simulink model "IMDriveSensor00"  (R2025a)
settings: Solver=FixedStepAuto  StartTime=0.0  StopTime=25  FixedStep=Ts  MaxStep=1e-3  RelTol=1e-3  EnableMultiTasking=on
PreLoadFcn:
  | IMDriveSensorData
values from neighbouring files (symbols this model uses):
  fn = 50    [IMDriveSensorData.m]
  Ibase = Pn/(1.5*Vbase)    [IMDriveSensorData.m]
  It1base = Pt/(1.5*Vt1base)    [IMDriveSensorData.m]
  Ki_id = 17.64    [IMDriveSensorData.m]
  Ki_ids = 207.58    [IMDriveSensorData.m]
  Ki_imr = 2790.51    [IMDriveSensorData.m]
  Ki_iq = 20.81    [IMDriveSensorData.m]
  Ki_iqs = 210.02    [IMDriveSensorData.m]
  Ki_vdc = 681.12    [IMDriveSensorData.m]
  Ki_wr = 3134.24    [IMDriveSensorData.m]
  Kp_id = 0.84    [IMDriveSensorData.m]
  Kp_ids = 1.08    [IMDriveSensorData.m]
  Kp_imr = 52.22    [IMDriveSensorData.m]
  Kp_iq = 0.99    [IMDriveSensorData.m]
  Kp_iqs = 1.08    [IMDriveSensorData.m]
  Kp_vdc = 3.54    [IMDriveSensorData.m]
  Kp_wr = 65.47    [IMDriveSensorData.m]
  Leq = (L1 + L2*(V1/V2)^2)/(Zt1base/wtbase)    [IMDriveSensorData.m]
  Lm = 1.36    [IMDriveSensorData.m]
  N = V2/V1    (= 1)    [IMDriveSensorData.m]
  p = 2    [IMDriveSensorData.m]
  Req = (R1 + R2*(V1/V2)^2)/Zt1base    [IMDriveSensorData.m]
  Tbase = Pn/(wbase/p)    (= 3.56507072526)    [IMDriveSensorData.m]
  Ts = 5e-6    (= 5e-06)    [IMDriveSensorData.m]
  Tsc = 1/(fsw*10)    (= 5e-05)    [IMDriveSensorData.m]
  Vbase = Vn/sqrt(3)*sqrt(2)    [IMDriveSensorData.m]
  Vt1base = V1/sqrt(3)*sqrt(2)    [IMDriveSensorData.m]
  wtbase = 2*pi*ft    (= 314.159265359)    [IMDriveSensorData.m]
  Xls = Lls*Zbase    [IMDriveSensorData.m]
undefined symbols (not defined in the file or in its folder): ee
libraries: nesl_utility x23, ee_lib x16, fl_lib x8, slpidlib x7, eeTransforms x4, eeGeneralControl x4, simulink x3, eePwmGeneratorTwoLevel x2, eeSinusoidalMeasurement x1, eeAsmFluxObserver x1, spsPLL3phLib x1
(part 1 of 2)
CloseFcn:
  | clear simlog_IMDriveSensor
  | clear logsout_IMDriveSensor
Description:
  | Three-Phase Asynchronous Drive with Sensor Control
settings Model: Creator=The MathWorks, Inc.  LastModifiedBy=vhovh
settings SolverCC: AlgebraicLoopSolver=TrustRegion  AutoInsertRateTranBlk=on
settings DataIOCC: MaxDataPoints=510000  SaveOperatingPoint=on  SaveFormat=StructureWithTime  SaveOutput=off  SaveTime=off  ReturnWorkspaceOutputs=off  SignalLoggingName=logsout_IMDriveSensor
settings OptimizationCC: ReuseModelBlockBuffer=off  ExpressionDepthLimit=2147483647.0  LifeSpan=inf
settings DebuggingCC: AlgebraicLoopMsg=error  UnderspecifiedInitializationDetection=Classic  MergeDetectMultiDrivingBlocksExec=none  SolverPrmCheckMsg=warning  MultiTaskRateTransMsg=warning  UnconnectedInputMsg=warning  UnconnectedOutputMsg=warning  UnconnectedLineMsg=warning  StateNameClashWarn=warning  SFUnexpectedBacktrackingDiag=warning  SFNoUnconditionalDefaultTransitionDiag=warning  SFExecutionAtInitializationDiag=none  ArithmeticOperatorsInVariantConditions=warning
settings HardwareCC: ProdBitPerPointer=32.0  ProdBitPerSizeT=32.0  ProdBitPerPtrDiffT=32.0  ProdLargestAtomicFloat=None  ProdIntDivRoundTo=Undefined  ProdEndianess=Unspecified  ProdWordSize=32.0  ProdHWDeviceType=32-bit Generic
settings ModelReferenceCC: EnableRefExpFcnMdlSchedulingChecks=on  PropagateSignalLabelsOutOfModel=off
settings SFSimCC: SimUseLocalCustomCode=off  CustomCodeUndefinedFunction=UseInterfaceOnly
settings RTWCC: RTWUseLocalCustomCode=off  GPUComputeCapability=3.5  DLArmComputeVersion=19.05
settings CodeAppCC: StateflowObjectComments=on
settings GRTTargetCC: TargetLangStandard=C89/C90 (ANSI)
settings ConfigComp: CovMetricSettings=dw  CovSaveCumulativeToWorkspaceVar=on  CovSaveSingleToWorkspaceVar=on  CovExternalEMLEnable=off  CovSFcnEnable=off
settings SimscapeCC: SimscapeLogType=all  SimscapeLogSimulationStatistics=on  SimscapeLogName=simlog_IMDriveSensor  SimscapeLogDecimation=5.0  SimscapeLogDataHistory=510000.0

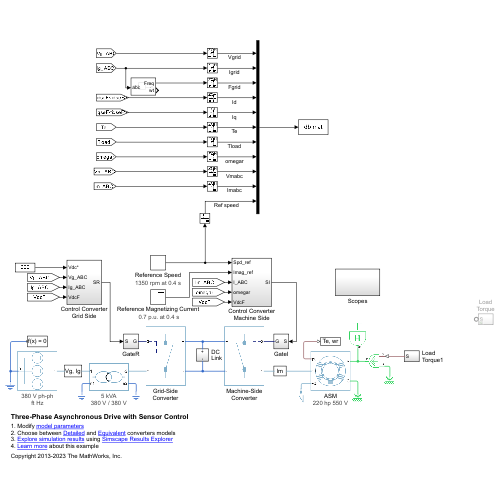
[thumbnail: Simulink's stored preview of the top-level diagram]
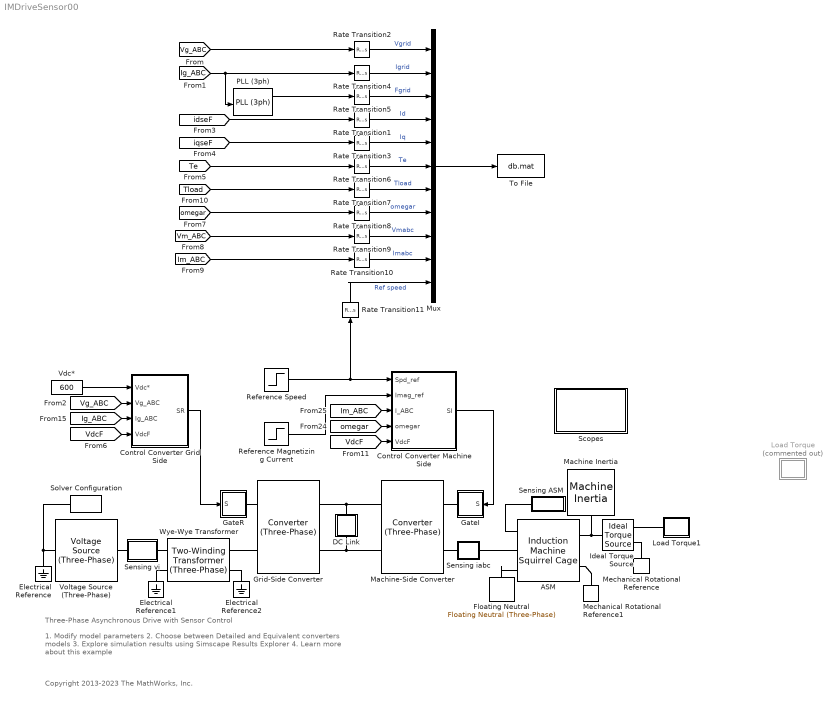
== system IMDriveSensor00 ==
  note: 1. Modify model parameters
      | 2. Choose between Detailed and Equivalent converters models
      | 3. Explore simulation results using Simscape Results Explorer
      | 4. Learn more about this example
  note: Three-Phase Asynchronous Drive with Sensor Control
  note: Copyright 2013-2023 The MathWorks, Inc.
  ASM : ee_lib/Electromechanical/Asynchronous/Induction Machine Squirrel Cage  port_option=ee.enum.threePhasePort.composite  SRated=Pn V*A  VRated=Vn V  FRated=fn Hz  nPolePairs=p  param_unit=ee.enum.unit.si  squirrel_cage=ee.enum.squirrelcage.Single  zero_sequence=ee.enum.park.zerosequence.include  initialization_option=ee.enum.asm.initialization.fluxvariables  Rs=Rss Ohm  Xls=Xls Ohm  pu_Rs=0.039  pu_Lls=0.194  Rrd=Rrr Ohm  Xlrd=Xlr Ohm  pu_Rrd=0.031  pu_Llrd=0.194  Rrd1=0.28 Ohm  Xlrd1=0.82 Ohm  Rrd2=0.28 Ohm  Xlrd2=0.82 Ohm  pu_Rrd1=0.0290  pu_Llrd1=0.0848  pu_Rrd2=0.0290  pu_Llrd2=0.0848  Xm=Xm Ohm  pu_Lm=1.36  X0=Xls Ohm  pu_L0=0.194  saturation_option=0  saturation_i=[0, 4, 9, 18, 25, 34, 50, 68, 95, 120] A  saturation_v=[0, 88, 154, 198, 220, 242, 264, 286, 308, 330] V  pu_saturation_i=[0, .176, .396, .792, 1.1, 1.496, 2.2, 2.992, 4.18, 5.28]  pu_saturation_v=[0, .4, .7, .9, 1, 1.1, 1.2, 1.3, 1.4, 1.4864]  connection_option=int32(ee.enum.Connection.delta)  angular_position_specify=off  angular_position_priority=None  angular_position=0 deg  angular_position_nominal_specify=off  angular_position_nominal_value=1  angular_position_nominal_unit=deg  pu_psids_specify=off  pu_psids_priority=None  pu_psids=0  pu_psids_nominal_specify=off  pu_psids_nominal_value=1  pu_psids_nominal_unit=1  pu_psiqs_specify=off  pu_psiqs_priority=None  pu_psiqs=0  pu_psiqs_nominal_specify=off  pu_psiqs_nominal_value=1  pu_psiqs_nominal_unit=1  pu_psi0s_specify=off  pu_psi0s_priority=None  pu_psi0s=0  pu_psi0s_nominal_specify=off  pu_psi0s_nominal_value=1  pu_psi0s_nominal_unit=1  pu_psidr_specify=off  pu_psidr_priority=None  pu_psidr=0  pu_psidr_nominal_specify=off  pu_psidr_nominal_value=1  pu_psidr_nominal_unit=1  pu_psiqr_specify=off  pu_psiqr_priority=None  pu_psiqr=0  pu_psiqr_nominal_specify=off  pu_psiqr_nominal_value=1  pu_psiqr_nominal_unit=1  pu_psidr1_specify=off  pu_psidr1_priority=None  pu_psidr1=0  pu_psidr1_nominal_specify=off  pu_psidr1_nominal_value=1  pu_psidr1_nominal_unit=1  pu_psiqr1_specify=off  pu_psiqr1_priority=None  pu_psiqr1=0  pu_psiqr1_nominal_specify=off  pu_psiqr1_nominal_value=1  pu_psiqr1_nominal_unit=1  pu_psidr2_specify=off  pu_psidr2_priority=None  pu_psidr2=0  pu_psidr2_nominal_specify=off  pu_psidr2_nominal_value=1  pu_psidr2_nominal_unit=1  pu_psiqr2_specify=off  pu_psiqr2_priority=None  pu_psiqr2=0  pu_psiqr2_nominal_specify=off  pu_psiqr2_nominal_value=1  pu_psiqr2_nominal_unit=1  psids_specify=off  psids_priority=None  psids=0 Wb  psids_nominal_specify=off  psids_nominal_value=1  psids_nominal_unit=Wb  psiqs_specify=off  psiqs_priority=None  psiqs=0 Wb  psiqs_nominal_specify=off  psiqs_nominal_value=1  psiqs_nominal_unit=Wb  psi0s_specify=off  psi0s_priority=None  psi0s=0 Wb  psi0s_nominal_specify=off  psi0s_nominal_value=1  psi0s_nominal_unit=Wb  psidr_specify=off  psidr_priority=None  psidr=0 Wb  psidr_nominal_specify=off  psidr_nominal_value=1  psidr_nominal_unit=Wb  psiqr_specify=off  psiqr_priority=None  psiqr=0 Wb  psiqr_nominal_specify=off  psiqr_nominal_value=1  psiqr_nominal_unit=Wb  psidr1_specify=off  psidr1_priority=None  psidr1=0 Wb  psidr1_nominal_specify=off  psidr1_nominal_value=1  psidr1_nominal_unit=Wb  psiqr1_specify=off  psiqr1_priority=None  psiqr1=0 Wb  psiqr1_nominal_specify=off  psiqr1_nominal_value=1  psiqr1_nominal_unit=Wb  psidr2_specify=off  psidr2_priority=None  psidr2=0 Wb  psidr2_nominal_specify=off  psidr2_nominal_value=1  psidr2_nominal_unit=Wb  psiqr2_specify=off  psiqr2_priority=None  psiqr2=0 Wb  psiqr2_nominal_specify=off  psiqr2_nominal_value=1  psiqr2_nominal_unit=Wb  slip_specify=off  slip_priority=None  slip=0  slip_nominal_specify=off  slip_nominal_value=1  slip_nominal_unit=1  real_power_generated_specify=off  real_power_generated_priority=None  real_power_generated=0 W  real_power_generated_nominal_specify=off  real_power_generated_nominal_value=1  real_power_generated_nominal_unit=W  mechanical_power_consumed_specify=off  mechanical_power_consumed_priority=None  mechanical_power_consumed=0 W  mechanical_power_consumed_nominal_specify=off  mechanical_power_consumed_nominal_value=1  mechanical_power_consumed_nominal_unit=W  Tmeas=298.15 K  alpha=3.93e-3 1/K  alpha_cage=4.4e-3 1/K  stator_thermal_mass=100 J/K  rotor_thermal_mass=200 J/K  temperatureA_specify=off  temperatureA_priority=High  temperatureA=25 degC  temperatureA_nominal_specify=off  temperatureA_nominal_value=1  temperatureA_nominal_unit=degC  temperatureB_specify=off  temperatureB_priority=High  temperatureB=25 degC  temperatureB_nominal_specify=off  temperatureB_nominal_value=1  temperatureB_nominal_unit=degC  temperatureC_specify=off  temperatureC_priority=High  temperatureC=25 degC  temperatureC_nominal_specify=off  temperatureC_nominal_value=1  temperatureC_nominal_unit=degC  temperatureR_specify=off  temperatureR_priority=High  temperatureR=25 degC  temperatureR_nominal_specify=off  temperatureR_nominal_value=1  temperatureR_nominal_unit=degC
      settings: AttributesFormatString=220 hp 550 V  InternalSimscapePortConfiguration="{\"Bottom\":[],\"Left\":[{\"id\":\"R\",\"label\":\"R\",\"type\":\"foundation.mechanical.rotational.rotational\"},{\"id\":\"C\",\"label\":\"C\",\"type\":\"foundation.mechanical.rotational.rotational\"}],\"Right\":[{\"id\":\"pu_output\",\"label\":\"pu\",\"type\":\"output\"},{\"id\":\"N1\",\"label\":\"~1\",\"type\":\"foundation.electrical.three_phase\"},{\"id\":\"N2\",\"label\":\"~2\",\"type\":\"foundation.electrical.three_phase\"}],\"Top\":[]}"
  Control Converter Grid Side : Subsystem
  Control Converter Machine Side : Subsystem
  DC Link : Subsystem
  Electrical Reference : fl_lib/Electrical/Electrical Elements/Electrical Reference
  Electrical Reference1 : fl_lib/Electrical/Electrical Elements/Electrical Reference
  Electrical Reference2 : fl_lib/Electrical/Electrical Elements/Electrical Reference
  Floating Neutral : ee_lib/Connectors & References/Floating Neutral (Three-Phase)  G_parasitic=1e-12 1/Ohm
      settings: InternalSimscapePortConfiguration="{\"Bottom\":[],\"Left\":[{\"id\":\"N\",\"label\":\"~\",\"type\":\"foundation.electrical.three_phase\"}],\"Right\":[],\"Top\":[]}"
  GateI : Subsystem
  GateR : Subsystem
  Grid-Side Converter : ee_lib/Semiconductors & Converters/Converters/Converter (Three-Phase)  port_option=ee.enum.threePhasePort.composite  fidelity_option=ee.enum.converters.fidelity.equivalent_pwm  device_type=3  showThermalPort=false  K=0  Vth=0.5 V  Vgt=1 V  Vgt_off=-1 V  Ih=1 A  Vf=0.8 V  Ron=0.001 Ohm  Rds=0.001 Ohm  Goff=1e-5 1/Ohm  Eon_scalar=22.86e-3 J  Eoff_scalar=17.14e-3 J  Eoff_natural_commutation=10e-3 J  Voff=300 V  Iout_scalar=600 A  onCurrentMeasDelay=0 s  useCurrentFromPreviousCycle=false  useVoltageFromPreviousCycle=false  diode_param=2  diode_Vf=0.8 V  diode_Ron=0.001 Ohm  diode_Goff=1e-5 1/Ohm  diode_C=50 nF  diode_iRM=-235 A  diode_iF=300 A  diode_idot=-50 A/us  diode_trr_param=1  diode_trr_factor=3  diode_trr=15 us  diode_Qrr=1.5e+3 s*uA  diode_rec_loss_model=ee.enum.diode.reverseRecoveryModel.fixed  diode_ErecVal=0 J  diode_scaleWithIandV=false  diode_ErecMat=zeros(2, 3) J  diode_TjrecVec=[298.15, 398.15] K  diode_IfrecVec=[.1, 1, 10] A  diode_IrecVal=10 A  diode_VrecVal=10 V  diode_tFilter=1 / 1000 / 100 s  thermal_network_parameterization=ee.enum.thermalNetworkTopology.external  Rth=[.08, .5] K/W  Rth_Cauer=[.08, .1, .5] K/W  Rth_Foster=[.08, .14, .22, .16] K/W  thermal_mass_parameterization=ee.enum.thermalNetwork.timeconstant  thermal_mass=[.01, .5] J/K  thermal_mass_Cauer=[.01, .1, .5] J/K  thermal_mass_Foster=[.001, .005, .05, .5] J/K  thermal_time_constant=[.001, .2] s  thermal_time_constant_Cauer=[.001, .1, .2] s  thermal_time_constant_Foster=[7e-05, .0007, .01, .08] s  thermal_mass_initial_temperatures=[25, 25] degC  thermal_mass_initial_temperatures_Cauer=[25, 25, 25] degC  junction_thermal_mass=0.01 J/K  Tvec_initial_Foster=[25, 25, 25, 25] degC  snubber_type=0  Cs=1e-5 F  Rs=1e-3 Ohm  Vce_loss=[0, 150, 300] V
  Ideal Torque Source : fl_lib/Mechanical/Mechanical Sources/Ideal Torque Source
  Load Torque : Subsystem  Commented=on
  Load Torque1 : Subsystem
  Machine Inertia : ee_lib/Electromechanical/Mechanical/Machine Inertia  SRated=Pn V*A  FRated=fn Hz  nPolePairs=p  inertia_option=2  J=27548 kg*m^2  H=H s*W/V/A  damper_option=2  D=39.0509 N*m/(rad/s)  pu_D=F  initialization_option=2  fMechanical0=60 Hz  fElectrical0=0 Hz
      settings: InternalSimscapePortConfiguration="{\"Bottom\":[],\"Left\":[{\"id\":\"R\",\"label\":\"R\",\"type\":\"foundation.mechanical.rotational.rotational\"}],\"Right\":[],\"Top\":[]}"
  Machine-Side Converter : ee_lib/Semiconductors & Converters/Converters/Converter (Three-Phase)  port_option=ee.enum.threePhasePort.composite  fidelity_option=ee.enum.converters.fidelity.equivalent_pwm  device_type=3  showThermalPort=false  K=0  Vth=0.5 V  Vgt=1 V  Vgt_off=-1 V  Ih=1 A  Vf=0.8 V  Ron=0.001 Ohm  Rds=0.001 Ohm  Goff=1e-5 1/Ohm  Eon_scalar=22.86e-3 J  Eoff_scalar=17.14e-3 J  Eoff_natural_commutation=10e-3 J  Voff=300 V  Iout_scalar=600 A  onCurrentMeasDelay=0 s  useCurrentFromPreviousCycle=false  useVoltageFromPreviousCycle=false  diode_param=2  diode_Vf=0.8 V  diode_Ron=0.001 Ohm  diode_Goff=1e-5 1/Ohm  diode_C=50 nF  diode_iRM=-235 A  diode_iF=300 A  diode_idot=-50 A/us  diode_trr_param=1  diode_trr_factor=3  diode_trr=15 us  diode_Qrr=1.5e+3 s*uA  diode_rec_loss_model=ee.enum.diode.reverseRecoveryModel.fixed  diode_ErecVal=0 J  diode_scaleWithIandV=false  diode_ErecMat=zeros(2, 3) J  diode_TjrecVec=[298.15, 398.15] K  diode_IfrecVec=[.1, 1, 10] A  diode_IrecVal=10 A  diode_VrecVal=10 V  diode_tFilter=1 / 1000 / 100 s  thermal_network_parameterization=ee.enum.thermalNetworkTopology.external  Rth=[.08, .5] K/W  Rth_Cauer=[.08, .1, .5] K/W  Rth_Foster=[.08, .14, .22, .16] K/W  thermal_mass_parameterization=ee.enum.thermalNetwork.timeconstant  thermal_mass=[.01, .5] J/K  thermal_mass_Cauer=[.01, .1, .5] J/K  thermal_mass_Foster=[.001, .005, .05, .5] J/K  thermal_time_constant=[.001, .2] s  thermal_time_constant_Cauer=[.001, .1, .2] s  thermal_time_constant_Foster=[7e-05, .0007, .01, .08] s  thermal_mass_initial_temperatures=[25, 25] degC  thermal_mass_initial_temperatures_Cauer=[25, 25, 25] degC  junction_thermal_mass=0.01 J/K  Tvec_initial_Foster=[25, 25, 25, 25] degC  snubber_type=0  Cs=1e-7 F  Rs=0.1 Ohm  Vce_loss=[0, 150, 300] V
  Mechanical Rotational Reference : fl_lib/Mechanical/Rotational Elements/Mechanical Rotational Reference
  Mechanical Rotational Reference1 : fl_lib/Mechanical/Rotational Elements/Mechanical Rotational Reference
  Mux : Mux  Inputs=11
  PLL (3ph) : spsPLL3phLib/PLL (3ph)  Fmin=45  Par_Init=[0, 60]  ParK=[180, 3200, 1]  TcD=1e-4  MaxRateChangeFreq=12  FilterCutOffFreq=25  Ts=0  AGC=on
  Rate Transition{1..11} (11 alike) : RateTransition  OutPortSampleTime=0.1
  Reference Magnetizing Current : Step  Time=0.4  After=0.7*1/Lm  SampleTime=Tsc
      settings: AttributesFormatString=0.7 p.u. at 0.4 s
  Reference Speed : Step  Time=0.4  After=1350  SampleTime=Tsc
      settings: AttributesFormatString=%<After> rpm at %<Time> s
  Scopes : Subsystem
  Sensing ASM : Subsystem
      mask Display: disp('Te, wr')
  Sensing iabc : Subsystem
      mask Display: disp('Im')
  Sensing vi : Subsystem
      mask Display: disp('Vg, Ig')
  Solver Configuration : nesl_utility/Solver Configuration  PhysicalDomain=network_engine_domain  SubClassName=solver  LeftPortType=input  RightPortType=generic  Tones=[]  Harmonics=[]  SimulateNoise=off  Profile=off  UseLocalSampling=off  EnableSwitchedLinearOptims=on  FrequencyDomain=off  UseCCode=off  RelTol=0.001  AbsTol=1e-06  MinStep=1e-09  ToWorkspace=off  RevertToSquareIcSolve=off  NumHomotopyIterations=100  PhasorMode=off  PhasorModeNumHarmonics=1  ConsistencySolver=NEWTON_FTOL  IndexReductionMethod=DerivativeReplacement  DoDC=off  ResidualTolerance=1e-09  ConsistencyTolSource=GLOBAL  ConsistencyAbsTol=0.001  ConsistencyRelTol=0.001  ConsistencyTolFactor=0.001  UseLocalSolver=on  LocalSolverChoice=NE_BACKWARD_EULER_ADVANCER  ResolveIndetEquations=on  FunctionEvalNumThread=1  LocalSolverSampleTime=Ts  DoFixedCost=on  MaxNonlinIter=5  MaxModeIter=2  ComputeImpulses=off  ImpulseIterations=2  LinearAlgebra=auto  LinearAlgebraNumThread=0  EquationFormulation=NE_TIME_EF  DelaysMemoryBudget=1024  AutomaticFiltering=on  FilteringTimeConstant=0.001  PartitionStorageMethod=AS_NEEDED  PartitionMemoryBudget=1024  PartitionMethod=FAST  MultibodyUseLocalSolver=off  MultibodyLocalSolverChoice=ODE1  MultibodyLocalSolverSampleTime=0.001
  To File : ToFile  Filename=db.mat  SaveFormat=Timeseries
  Vdc* : Constant  Value=600
  Voltage Source (Three-Phase) : ee_lib/Sources/Voltage Source (Three-Phase)  vline_rms=380 V  shift=0 deg  freq=ft Hz  impedance_option=0  SShortCircuit=1e6 V*A  XR=15  R=0.01 Ohm  L=3.97e-4 H  harmonic_option=0  harmonic_orders=[5.0, 7.0, 11.0, 13.0]  harmonic_ratios=[0.1, 0.1, 0.1, 0.1]  G_parasitic=0 1/Ohm  I_specify=off  I_priority=None  I=[ 0 0 0 ] A  I_nominal_specify=off  I_nominal_value=1  I_nominal_unit=A
      settings: AttributesFormatString=|
      | %<vline_rms> %<vline_rms_unit> ph-ph
      | %<freq> %<freq_unit>
  Wye-Wye Transformer : ee_lib/Passive/Transformers/Two-Winding Transformer (Three-Phase)  SRated=Pt V*A  FRated=ft Hz  Winding1Connection=ee.enum.windingconnection.Yn  VRated1=V1 V  Winding2Connection=ee.enum.windingconnection.Yn  VRated2=V2 V  CoreType=ee.enum.coretype.threelimb  pu_Rw1=0.01  pu_Rw2=0.01  leakage_reactance_option=ee.enum.transformer_leakage.include  pu_Xl1=L1pu  pu_Xl2=L2pu  magnetizing_resistance_option=ee.enum.transformer_magnetizingResistance.include  pu_Rm=500  magnetizing_reactance_option=ee.enum.transformer_magnetizingReactance.include  saturation_option=ee.enum.transformer_saturation.exclude  pu_Xm=500  current_data=[0, .002, 1, 2]  magnetic_flux_data=[0, 1.2, 1.5, 1.51]  pu_X0=0.5  i1_specify=off  i1_priority=None  i1=[ 0 0 0 ] A  i1_nominal_specify=off  i1_nominal_value=1  i1_nominal_unit=A  i2_specify=off  i2_priority=None  i2=[ 0 0 0 ] A  i2_nominal_specify=off  i2_nominal_value=1  i2_nominal_unit=A  phi_specify=off  phi_priority=None  phi=[ 0 0 0 ]  phi_nominal_specify=off  phi_nominal_value=1  phi_nominal_unit=1  power_dissipated_specify=off  power_dissipated_priority=None  power_dissipated=0 W  power_dissipated_nominal_specify=off  power_dissipated_nominal_value=1  power_dissipated_nominal_unit=W
      settings: InternalSimscapePortConfiguration="{\"Bottom\":[],\"Left\":[{\"id\":\"N1\",\"label\":\"~1\",\"type\":\"foundation.electrical.three_phase\"},{\"id\":\"n1\",\"label\":\"n1\",\"type\":\"foundation.electrical.electrical\"}],\"Right\":[{\"id\":\"N2\",\"label\":\"~2\",\"type\":\"foundation.electrical.three_phase\"},{\"id\":\"n2\",\"label\":\"n2\",\"type\":\"foundation.electrical.electrical\"}],\"Top\":[]}"
      settings: AttributesFormatString=|
      | 5 kVA
      | 380 V / 380 V
  wires:
  Control Converter Grid Side/1(SR) -> GateR/1(S)
  Control Converter Machine Side/1(SI) -> GateI/1(S)
  Reference Speed/1 -> Rate Transition11/1, Control Converter Machine Side/1(Spd_ref)
  Reference Magnetizing Current/1 -> Control Converter Machine Side/2(Imag_ref)
  Vdc*/1 -> Control Converter Grid Side/1(Vdc*)
  [Vg_ABC] -> Control Converter Grid Side/2(Vg_ABC)
  [Ig_ABC] -> Control Converter Grid Side/3(Ig_ABC)
  [VdcF] -> Control Converter Grid Side/4(VdcF)
  [Im_ABC] -> Control Converter Machine Side/3(I_ABC)
  [omegar] -> Control Converter Machine Side/4(omegar)
  [VdcF] -> Control Converter Machine Side/5(VdcF)
  [Vg_ABC] -> Rate Transition2/1
  [Ig_ABC] -> PLL (3ph)/1, Rate Transition4/1
  PLL (3ph)/1 -> Rate Transition5/1
  [Te] -> Rate Transition6/1
  [Tload] -> Rate Transition7/1
  [omegar] -> Rate Transition8/1
  [Vm_ABC] -> Rate Transition9/1
  [Im_ABC] -> Rate Transition10/1
  Mux/1 -> To File/1
  [iqseF] -> Rate Transition3/1
  [idseF] -> Rate Transition1/1
  Rate Transition2/1 -> Mux/1  "Vgrid"
  Rate Transition4/1 -> Mux/2  "Igrid"
  Rate Transition5/1 -> Mux/3  "Fgrid"
  Rate Transition1/1 -> Mux/4  "Id"
  Rate Transition3/1 -> Mux/5  "Iq"
  Rate Transition6/1 -> Mux/6  "Te"
  Rate Transition7/1 -> Mux/7  "Tload"
  Rate Transition8/1 -> Mux/8  "omegar"
  Rate Transition9/1 -> Mux/9  "Vmabc"
  Rate Transition10/1 -> Mux/10  "Imabc"
  Rate Transition11/1 -> Mux/11  "Ref speed"
  connections:
  Electrical Reference/LConn1 -- Solver Configuration/RConn1 -- Voltage Source (Three-Phase)/LConn1
  Sensing vi/LConn1 -- Voltage Source (Three-Phase)/RConn1
  Sensing vi/RConn1 -- Wye-Wye Transformer/LConn1
  Electrical Reference1/LConn1 -- Wye-Wye Transformer/LConn2
  Wye-Wye Transformer/RConn2 -- Electrical Reference2/LConn1
  Grid-Side Converter/LConn2 -- Wye-Wye Transformer/RConn1
  Grid-Side Converter/RConn1 -- DC Link/LConn1 -- Machine-Side Converter/RConn1
  Grid-Side Converter/RConn2 -- DC Link/RConn1 -- Machine-Side Converter/RConn2
  Sensing iabc/LConn1 -- Machine-Side Converter/LConn2
  ASM/RConn2 -- Sensing iabc/RConn1
  ASM/LConn1 -- Machine Inertia/LConn1 -- Ideal Torque Source/LConn1
  Mechanical Rotational Reference/LConn1 -- Ideal Torque Source/RConn2
  GateR/RConn1 -- Grid-Side Converter/LConn1
  GateI/RConn1 -- Machine-Side Converter/LConn1
  Floating Neutral/LConn1 -- ASM/RConn3
  Mechanical Rotational Reference1/LConn1 -- ASM/LConn2
  Load Torque1/RConn1 -- Ideal Torque Source/RConn1
  ASM/RConn1 -- Sensing ASM/RConn1

== system IMDriveSensor00/Control Converter Grid Side ==
  Vdc* : Inport
  Vg_ABC : Inport  Port=2
  Ig_ABC : Inport  Port=3
  VdcF : Inport  Port=4
  Control : Subsystem
  Measurements : Subsystem
  SR : Outport  VectorParamsAs1DForOutWhenUnconnected=off
  wires:
  Vdc*/1 -> Control/1(Vdc)
  VdcF/1 -> Control/2(VdcF)
  Control/1(SR) -> SR/1
  Vg_ABC/1 -> Measurements/1(Vg_ABC)
  Ig_ABC/1 -> Measurements/2(Ig_ABC)
  Measurements/1(omega) -> Control/3(omega)
  Measurements/2(Vg) -> Control/4(Vg)
  Measurements/3(idF) -> Control/5(idF)
  Measurements/4(theta) -> Control/6(theta)
  Measurements/5(iqF) -> Control/7(iqF)

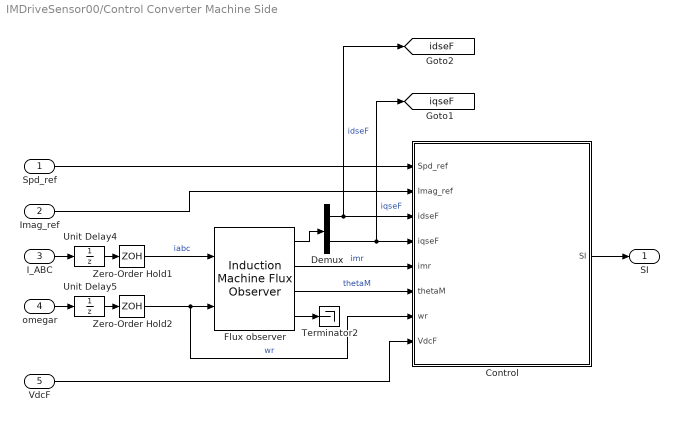
== system IMDriveSensor00/Control Converter Machine Side ==
  Spd_ref : Inport
  Imag_ref : Inport  Port=2
  I_ABC : Inport  Port=3
  omegar : Inport  Port=4
  VdcF : Inport  Port=5
  Control : Subsystem
  Demux : Demux  Outputs=2
  Flux observer : eeAsmFluxObserver/Induction Machine Flux Observer  fn=fn  Rr=Rr  Llr=Llr  Lm=Lm  Tc=1e-4  Ts=Tsc
  Terminator2 : Terminator
  Unit Delay4 : UnitDelay  SampleTime=Ts  HasFrameUpgradeWarning=on
  Unit Delay5 : UnitDelay  SampleTime=Ts  HasFrameUpgradeWarning=on
  Zero-Order Hold1 : ZeroOrderHold  SampleTime=Tsc
  Zero-Order Hold2 : ZeroOrderHold  SampleTime=Tsc
  SI : Outport  VectorParamsAs1DForOutWhenUnconnected=off
  tag scope: idseF=global, iqseF=global
  wires:
  Zero-Order Hold1/1 -> Flux observer/1  "iabc"
  Flux observer/1 -> Demux/1
  Flux observer/4 -> Terminator2/1
  Imag_ref/1 -> Control/2(Imag_ref)
  Demux/1 -> [idseF], Control/3(idseF)  "idseF"
  Demux/2 -> [iqseF], Control/4(iqseF)  "iqseF"
  Flux observer/2 -> Control/5(imr)  "imr"
  Flux observer/3 -> Control/6(thetaM)  "thetaM"
  Zero-Order Hold2/1 -> Control/7(wr), Flux observer/2  "wr"
  Spd_ref/1 -> Control/1(Spd_ref)
  VdcF/1 -> Control/8(VdcF)
  Control/1(SI) -> SI/1
  Unit Delay5/1 -> Zero-Order Hold2/1
  omegar/1 -> Unit Delay5/1
  Unit Delay4/1 -> Zero-Order Hold1/1
  I_ABC/1 -> Unit Delay4/1

== system IMDriveSensor00/DC Link ==
  C : fl_lib/Electrical/Electrical Elements/Capacitor  c=5000e-6 F  r=2e-3 Ohm  g=0 1/Ohm  i_specify=off  i_priority=None  i=0 A  i_nominal_specify=off  i_nominal_value=1  i_nominal_unit=A  v_specify=off  v_priority=None  v=0 V  v_nominal_specify=off  v_nominal_value=1  v_nominal_unit=V  vc_specify=on  vc_priority=None  vc=0 V  vc_nominal_specify=off  vc_nominal_value=1  vc_nominal_unit=V
  Sensing Vdc : Subsystem
      mask Display: disp('Vdc')
  + : PMIOPort  Side=Left
  - : PMIOPort  Port=2  Side=Right
  connections:
  C/RConn1 -- -/RConn1 -- Sensing Vdc/RConn1
  C/LConn1 -- Sensing Vdc/LConn1 -- +/RConn1

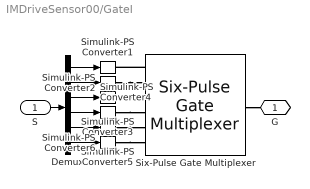
== system IMDriveSensor00/GateI ==
  S : Inport
  Demux : Demux  Outputs=6
  Simulink-PS Converter{1..6} (6 alike) : nesl_utility/Simulink-PS Converter  PhysicalDomain=network_engine_domain  SubClassName=ps_input  LeftPortType=input  RightPortType=output  PseudoPeriodic=off  Frequencies=[]  NoiseDistribution=none  NoiseParameters=[]  Unit=1  AffineConversion=off  FilteringAndDerivatives=zero  SimscapeFilterOrder=1  InputFilterTimeConstant=0.001  UdotUserProvided=1
  Six-Pulse Gate Multiplexer : ee_lib/Semiconductors & Converters/Converters/Six-Pulse Gate Multiplexer  port_option=ee.enum.controlport.ps
  G : PMIOPort  Side=Right
  wires:
  Demux/3 -> Simulink-PS Converter3/1
  Demux/6 -> Simulink-PS Converter6/1
  Demux/5 -> Simulink-PS Converter5/1
  S/1 -> Demux/1
  Demux/2 -> Simulink-PS Converter2/1
  Demux/1 -> Simulink-PS Converter1/1
  Demux/4 -> Simulink-PS Converter4/1
  connections:
  Six-Pulse Gate Multiplexer/RConn1 -- G/RConn1
  Six-Pulse Gate Multiplexer/LConn1 -- Simulink-PS Converter1/RConn1
  Simulink-PS Converter5/RConn1 -- Six-Pulse Gate Multiplexer/LConn5
  Simulink-PS Converter6/RConn1 -- Six-Pulse Gate Multiplexer/LConn6
  Simulink-PS Converter3/RConn1 -- Six-Pulse Gate Multiplexer/LConn3
  Simulink-PS Converter2/RConn1 -- Six-Pulse Gate Multiplexer/LConn2
  Simulink-PS Converter4/RConn1 -- Six-Pulse Gate Multiplexer/LConn4

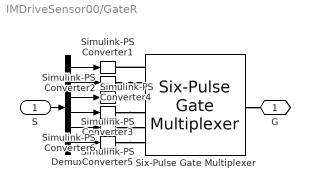
== system IMDriveSensor00/GateR ==
  S : Inport
  Demux : Demux  Outputs=6
  Simulink-PS Converter{1..6} (6 alike) : nesl_utility/Simulink-PS Converter  PhysicalDomain=network_engine_domain  SubClassName=ps_input  LeftPortType=input  RightPortType=output  PseudoPeriodic=off  Frequencies=[]  NoiseDistribution=none  NoiseParameters=[]  Unit=1  AffineConversion=off  FilteringAndDerivatives=zero  SimscapeFilterOrder=1  InputFilterTimeConstant=0.001  UdotUserProvided=1
  Six-Pulse Gate Multiplexer : ee_lib/Semiconductors & Converters/Converters/Six-Pulse Gate Multiplexer  port_option=ee.enum.controlport.ps
  G : PMIOPort  Side=Right
  wires:
  Demux/4 -> Simulink-PS Converter4/1
  Demux/1 -> Simulink-PS Converter1/1
  Demux/2 -> Simulink-PS Converter2/1
  S/1 -> Demux/1
  Demux/5 -> Simulink-PS Converter5/1
  Demux/6 -> Simulink-PS Converter6/1
  Demux/3 -> Simulink-PS Converter3/1
  connections:
  Simulink-PS Converter4/RConn1 -- Six-Pulse Gate Multiplexer/LConn4
  Simulink-PS Converter2/RConn1 -- Six-Pulse Gate Multiplexer/LConn2
  Simulink-PS Converter3/RConn1 -- Six-Pulse Gate Multiplexer/LConn3
  Simulink-PS Converter6/RConn1 -- Six-Pulse Gate Multiplexer/LConn6
  Simulink-PS Converter5/RConn1 -- Six-Pulse Gate Multiplexer/LConn5
  Six-Pulse Gate Multiplexer/LConn1 -- Simulink-PS Converter1/RConn1
  Six-Pulse Gate Multiplexer/RConn1 -- G/RConn1

== system IMDriveSensor00/Load Torque ==
  -Tbase1 : Constant  Value=-1  SampleTime=Ts
  ">= 0.5 " : Switch  Threshold=0.5  SaturateOnIntegerOverflow=off  InputSameDT=off
  Gain : Gain  Gain=-Tbase
  Simulink-PS Converter : nesl_utility/Simulink-PS Converter  PhysicalDomain=network_engine_domain  SubClassName=ps_input  LeftPortType=input  RightPortType=output  PseudoPeriodic=off  Frequencies=[]  NoiseDistribution=none  NoiseParameters=[]  Unit=1  AffineConversion=off  FilteringAndDerivatives=zero  SimscapeFilterOrder=1  InputFilterTimeConstant=0.001  UdotUserProvided=1
  Step1 : Step  Time=2.1  SampleTime=Ts
      settings: AttributesFormatString=1 at 2.1 s
  Tbase1 : Step  Time=1.6  SampleTime=Ts
      settings: AttributesFormatString=1 p.u. at 1.6 s
  S : PMIOPort  Side=Right
  tag scope: Tload=global
  wires:
  ">= 0.5 "/1 -> [Tload], Gain/1
  -Tbase1/1 -> ">= 0.5 "/1
  Step1/1 -> ">= 0.5 "/2
  Gain/1 -> Simulink-PS Converter/1
  Tbase1/1 -> ">= 0.5 "/3
  connections:
  Simulink-PS Converter/RConn1 -- S/RConn1

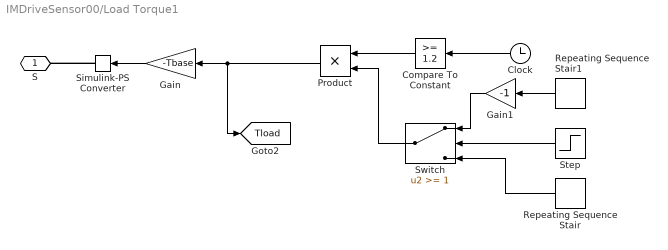
== system IMDriveSensor00/Load Torque1 ==
  Clock : Clock
  Compare To Constant : simulink/Logic and Bit Operations/Compare To Constant  relop=>=  const=1.2  OutDataTypeStr=boolean
  Gain : Gain  Gain=-Tbase
  Gain1 : Gain  Gain=-1
  Product : Product
  Repeating Sequence Stair : simulink/Sources/Repeating Sequence Stair  OutValues=[0 0 0.1 0.2 0.3 0.4 0.5 0.6 0.7 0.8 0.9 1 1.1 1.2 0 0.5 0 0.7 0 1].'  tsamp=0.5  OutMin=[]  OutMax=[]  OutDataTypeStr=double  OutputDataTypeScalingMode=double  OutDataType=fixdt(0,8)  ConRadixGroup=Best Precision: Vector-wise  OutScaling=2^-12
  Repeating Sequence Stair1 : simulink/Sources/Repeating Sequence Stair  OutValues=[0 0 0.1 0.2 0.3 0.4 0.5 0.6 0.7 0.8 0.9 1 1.1 1.2 0 0.5 0 0.7 0 1].'  tsamp=0.5  OutMin=[]  OutMax=[]  OutDataTypeStr=double  OutputDataTypeScalingMode=double  OutDataType=fixdt(0,8)  ConRadixGroup=Best Precision: Vector-wise  OutScaling=2^-12
  Simulink-PS Converter : nesl_utility/Simulink-PS Converter  PhysicalDomain=network_engine_domain  SubClassName=ps_input  LeftPortType=input  RightPortType=output  PseudoPeriodic=off  Frequencies=[]  NoiseDistribution=none  NoiseParameters=[]  Unit=1  AffineConversion=off  FilteringAndDerivatives=zero  SimscapeFilterOrder=1  InputFilterTimeConstant=0.001  UdotUserProvided=1
  Step : Step  Time=11  SampleTime=0
  Switch : Switch  Threshold=1  SaturateOnIntegerOverflow=off  InputSameDT=off
  S : PMIOPort  Side=Right
  tag scope: Tload=global
  wires:
  Gain/1 -> Simulink-PS Converter/1
  Compare To Constant/1 -> Product/1
  Clock/1 -> Compare To Constant/1
  Product/1 -> Gain/1, [Tload]
  Repeating Sequence Stair1/1 -> Gain1/1
  Step/1 -> Switch/2
  Switch/1 -> Product/2
  Gain1/1 -> Switch/1
  Repeating Sequence Stair/1 -> Switch/3
  connections:
  Simulink-PS Converter/RConn1 -- S/RConn1

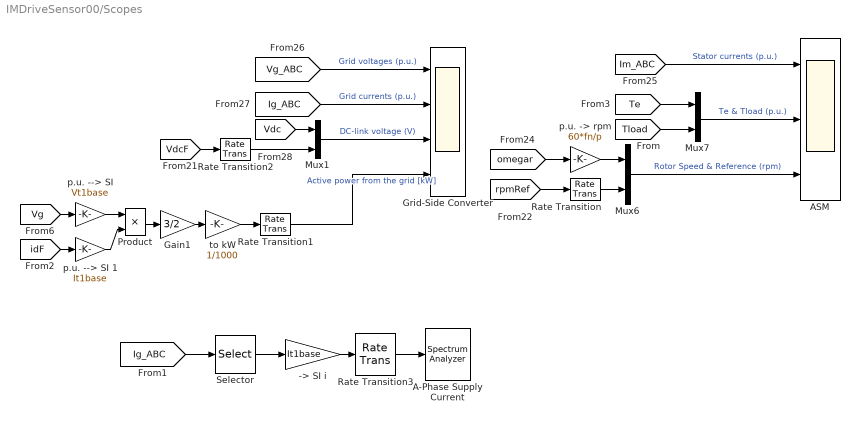
== system IMDriveSensor00/Scopes ==
  -> SI i : Gain  Gain=It1base
  A-Phase Supply Current : SpectrumAnalyzer  WindowPosition=[-1289.000000,581.000000,1030.000000,450.000000,]  Visible=on  ScopeFrameLocation=window  SpectrumType=RMS  Method=Welch  PlotAsTwoSidedSpectrum=off  AxesScaling=Manual  RBWSource=Property  RBW=9  Span=5000  CenterFrequency=2500  StartFrequency=0  OverlapPercent=90  AveragingMethod=Running  SpectrumUnits=Vrms  YLimits=[-0.1135 1.0222]  AllowFFTLengthLessThanSamplesPerUpdate=on
  ASM : Scope  NumInputPorts=3
      settings: ActiveDisplayYMinimum=-2.631713451080445  ActiveDisplayYMaximum=2.6311943378029681  DataLoggingVariableName=ScopeData2
  Gain1 : Gain  Gain=3/2
  Grid-Side Converter : Scope  NumInputPorts=4
      settings: ActiveDisplayYMinimum=-1.2499999999999998  ActiveDisplayYMaximum=1.2499999999999998
  Mux1 : Mux  Inputs=2
  Mux6 : Mux  Inputs=2
  Mux7 : Mux  Inputs=2
  Product : Product
  Rate Transition : RateTransition
  Rate Transition1 : RateTransition
  Rate Transition2 : RateTransition
  Rate Transition3 : RateTransition  OutPortSampleTime=1e-4
  Selector : Selector  InputPortWidth=3  IndexOptions=Index vector (dialog)  Indices=1  OutputSizes=1
  p.u. --> SI : Gain  Gain=Vt1base
  p.u. --> SI 1 : Gain  Gain=It1base
  "p.u. -> rpm" : Gain  Gain=60*fn/p
  to kW : Gain  Gain=1/1000
  wires:
  [VdcF] -> Rate Transition2/1
  [Im_ABC] -> ASM/1  "Stator currents (p.u.)"
  Mux7/1 -> ASM/2  "Te & Tload (p.u.)"
  [Tload] -> Mux7/2
  Mux6/1 -> ASM/3  "Rotor Speed & Reference (rpm)"
  [Vdc] -> Mux1/1
  Mux1/1 -> Grid-Side Converter/3  "DC-link voltage (V)"
  [Vg_ABC] -> Grid-Side Converter/1  "Grid voltages (p.u.)"
  [rpmRef] -> Rate Transition/1
  "p.u. -> rpm"/1 -> Mux6/1
  [Ig_ABC] -> Grid-Side Converter/2  "Grid currents (p.u.)"
  to kW/1 -> Rate Transition1/1
  [Te] -> Mux7/1
  [omegar] -> "p.u. -> rpm"/1
  p.u. --> SI/1 -> Product/1
  Gain1/1 -> to kW/1
  p.u. --> SI 1/1 -> Product/2
  Product/1 -> Gain1/1
  [idF] -> p.u. --> SI 1/1
  [Vg] -> p.u. --> SI/1
  Rate Transition/1 -> Mux6/2
  Rate Transition1/1 -> Grid-Side Converter/4  "Active power from the grid [kW]"
  Rate Transition2/1 -> Mux1/2
  [Ig_ABC] -> Selector/1
  Selector/1 -> -> SI i/1
  Rate Transition3/1 -> A-Phase Supply Current/1
  -> SI i/1 -> Rate Transition3/1

== system IMDriveSensor00/Sensing ASM ==
  Electromagnetic torque : ee_lib/Electromechanical/Asynchronous/Induction Machine Measurement  output_idx=1
      settings: InternalSimscapePortConfiguration="{\"Bottom\":[],\"Left\":[{\"id\":\"pu_input\",\"label\":\"pu\",\"type\":\"input\"}],\"Right\":[{\"id\":\"pu_output\",\"label\":\"o\",\"type\":\"output\"}],\"Top\":[]}"
  PS-Simulink Converter1 : nesl_utility/PS-Simulink Converter  PhysicalDomain=network_engine_domain  SubClassName=ps_output  LeftPortType=input  RightPortType=output  PseudoPeriodic=off  Frequencies=[]  VectorFormat=1-D array  Unit=1  AffineConversion=off
  PS-Simulink Converter2 : nesl_utility/PS-Simulink Converter  PhysicalDomain=network_engine_domain  SubClassName=ps_output  LeftPortType=input  RightPortType=output  PseudoPeriodic=off  Frequencies=[]  VectorFormat=1-D array  Unit=1  AffineConversion=off
  Rotor speed : ee_lib/Electromechanical/Asynchronous/Induction Machine Measurement  output_idx=2
      settings: InternalSimscapePortConfiguration="{\"Bottom\":[],\"Left\":[{\"id\":\"pu_input\",\"label\":\"pu\",\"type\":\"input\"}],\"Right\":[{\"id\":\"pu_output\",\"label\":\"o\",\"type\":\"output\"}],\"Top\":[]}"
  pu : PMIOPort  Side=Right
  tag scope: Te=global, omegar=global
  wires:
  PS-Simulink Converter2/1 -> [omegar]
  PS-Simulink Converter1/1 -> [Te]
  connections:
  Electromagnetic torque/LConn1 -- Rotor speed/LConn1 -- pu/RConn1
  PS-Simulink Converter1/LConn1 -- Electromagnetic torque/RConn1
  PS-Simulink Converter2/LConn1 -- Rotor speed/RConn1

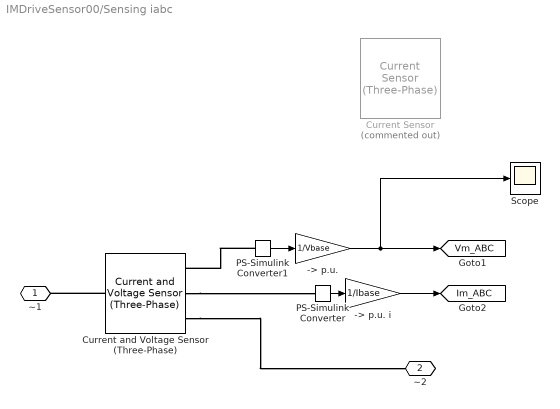
== system IMDriveSensor00/Sensing iabc ==
  -> p.u. : Gain  Gain=1/Vbase
  -> p.u. i : Gain  Gain=1/Ibase
  Current Sensor : ee_lib/Sensors & Transducers/Current Sensor (Three-Phase)  Commented=on
  Current and Voltage Sensor (Three-Phase) : ee_lib/Sensors & Transducers/Current and Voltage Sensor (Three-Phase)  vMeasurementType=ee.enum.vmeasurement.ll  outputUnit=ee.enum.unit.si  SRated=100e6 A*V  VRated=24e3 V  I_specify=off  I_priority=None  I=[0, 0, 0] A  I_nominal_specify=off  I_nominal_value=1  I_nominal_unit=A  V_specify=off  V_priority=None  V=[0, 0, 0] V  V_nominal_specify=off  V_nominal_value=1  V_nominal_unit=V
      settings: InternalSimscapePortConfiguration="{\"Bottom\":[],\"Left\":[{\"id\":\"N1\",\"label\":\"~1\",\"type\":\"foundation.electrical.three_phase\"}],\"Right\":[{\"id\":\"V_output\",\"label\":\"V\",\"type\":\"output\"},{\"id\":\"I_output\",\"label\":\"I\",\"type\":\"output\"},{\"id\":\"N2\",\"label\":\"~2\",\"type\":\"foundation.electrical.three_phase\"}],\"Top\":[]}"
  PS-Simulink Converter : nesl_utility/PS-Simulink Converter  PhysicalDomain=network_engine_domain  SubClassName=ps_output  LeftPortType=input  RightPortType=output  PseudoPeriodic=off  Frequencies=[]  VectorFormat=1-D array  Unit=1  AffineConversion=off
  PS-Simulink Converter1 : nesl_utility/PS-Simulink Converter  PhysicalDomain=network_engine_domain  SubClassName=ps_output  LeftPortType=input  RightPortType=output  PseudoPeriodic=off  Frequencies=[]  VectorFormat=1-D array  Unit=1  AffineConversion=off
  Scope : Scope
      settings: ActiveDisplayYMinimum=-2.4318306446613431  ActiveDisplayYMaximum=2.4318306446613431  DataLoggingVariableName=ScopeData3
  ~1 : PMIOPort  Side=Left
  ~2 : PMIOPort  Port=2  Side=Right
  tag scope: Im_ABC=global, Vm_ABC=global
  wires:
  PS-Simulink Converter/1 -> -> p.u. i/1
  -> p.u. i/1 -> [Im_ABC]
  -> p.u./1 -> Scope/1, [Vm_ABC]
  PS-Simulink Converter1/1 -> -> p.u./1
  connections:
  Current and Voltage Sensor (Three-Phase)/LConn1 -- ~1/RConn1
  Current and Voltage Sensor (Three-Phase)/RConn2 -- PS-Simulink Converter/LConn1
  Current and Voltage Sensor (Three-Phase)/RConn3 -- ~2/RConn1
  PS-Simulink Converter1/LConn1 -- Current and Voltage Sensor (Three-Phase)/RConn1

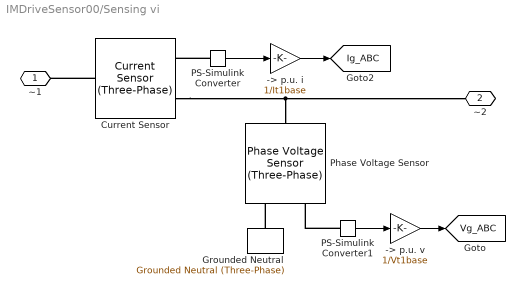
== system IMDriveSensor00/Sensing vi ==
  -> p.u. i : Gain  Gain=1/It1base
  -> p.u. v : Gain  Gain=1/Vt1base
  Current Sensor : ee_lib/Sensors & Transducers/Current Sensor (Three-Phase)
  Grounded Neutral : ee_lib/Connectors & References/Grounded Neutral (Three-Phase)
  PS-Simulink Converter : nesl_utility/PS-Simulink Converter  PhysicalDomain=network_engine_domain  SubClassName=ps_output  LeftPortType=input  RightPortType=output  PseudoPeriodic=off  Frequencies=[]  VectorFormat=1-D array  Unit=1  AffineConversion=off
  PS-Simulink Converter1 : nesl_utility/PS-Simulink Converter  PhysicalDomain=network_engine_domain  SubClassName=ps_output  LeftPortType=input  RightPortType=output  PseudoPeriodic=off  Frequencies=[]  VectorFormat=1-D array  Unit=1  AffineConversion=off
  Phase Voltage Sensor : ee_lib/Sensors & Transducers/Phase Voltage Sensor (Three-Phase)
  ~1 : PMIOPort  Side=Left
  ~2 : PMIOPort  Port=2  Side=Right
  tag scope: Ig_ABC=global, Vg_ABC=global
  wires:
  -> p.u. i/1 -> [Ig_ABC]
  PS-Simulink Converter1/1 -> -> p.u. v/1
  PS-Simulink Converter/1 -> -> p.u. i/1
  -> p.u. v/1 -> [Vg_ABC]
  connections:
  PS-Simulink Converter1/LConn1 -- Phase Voltage Sensor/RConn1
  Current Sensor/RConn2 -- Phase Voltage Sensor/LConn1 -- ~2/RConn1
  PS-Simulink Converter/LConn1 -- Current Sensor/RConn1
  Grounded Neutral/LConn1 -- Phase Voltage Sensor/RConn2
  Current Sensor/LConn1 -- ~1/RConn1

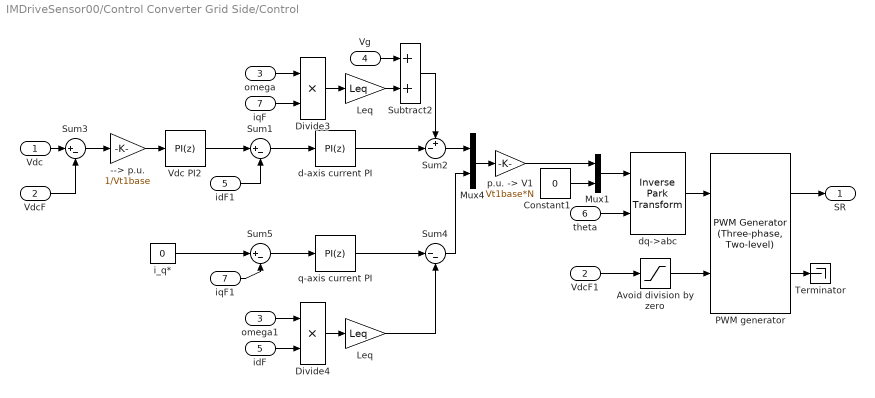
== system IMDriveSensor00/Control Converter Grid Side/Control ==
  Vdc : Inport
  VdcF : Inport  Port=2
  omega : Inport  Port=3
  Vg : Inport  Port=4
  idF : Inport  Port=5
  theta : Inport  Port=6
  iqF : Inport  Port=7
  --> p.u. : Gain  Gain=1/Vt1base
  Avoid division by zero : Saturate  UpperLimit=1e6  LowerLimit=10
  Constant1 : Constant  Value=0  SampleTime=Tsc
  Divide3 : Product  Inputs=**
  Divide4 : Product  Inputs=**
  Leq : Gain  Gain=Leq
  "Leq " : Gain  Gain=Leq
  Mux1 : Mux  Inputs=2
  Mux4 : Mux  Inputs=2
  PWM generator : eePwmGeneratorTwoLevel/PWM Generator (Three-phase, Two-level)  PWMMode=Continuous PWM (CPWM)  CPWMMode=SPWM: sinusoidal PWM  DPWMMode=60 DPWM: 60 degree discontinuous PWM  fsw=fsw  Ts=Ts
  Subtract2 : Sum
  Sum1 : Sum  Inputs=|+-
  Sum2 : Sum  Inputs=+-|
  Sum3 : Sum  Inputs=|+-
  Sum4 : Sum  Inputs=|--
  Sum5 : Sum  Inputs=|+-
  Terminator : Terminator
  Vdc PI2 : slpidlib/PID Controller  Controller=PI  Form=Parallel  TimeDomain=Discrete-time  UseExternalTs=off  SampleTime=Tsc  IntegratorMethod=Forward Euler  FilterMethod=Forward Euler  ControllerParametersSource=internal  P=Kp_vdc  I=Ki_vdc  UseKiTs=off  D=0  UseExternalDerivativeSource=off  N=100  UseFilter=on  TunerSelectOption=Transfer Function Based (PID Tuner App)  InitialConditionSource=internal  InitialConditionForIntegrator=0  InitialConditionForFilter=0  DifferentiatorICPrevScaledInput=0  ExternalReset=none  TrackingMode=off  Kt=1  LimitOutput=on  SatLimitsSource=internal  UpperSaturationLimit=2  LowerSaturationLimit=-2  LinearizeAsGain=on  AntiWindupMode=back-calculation  Kb=1000  LimitIntegrator=off  UpperIntegratorSaturationLimit=inf  LowerIntegratorSaturationLimit=-inf  POutMin=[]  POutMax=[]  IOutMin=[]  IOutMax=[]  DOutMin=[]  DOutMax=[]  NOutMin=[]  NOutMax=[]  SumOutMin=[]  SumOutMax=[]  SaturationOutMin=[]  SaturationOutMax=[]  PParamMin=[]  PParamMax=[]  IParamMin=[]  IParamMax=[]  DParamMin=[]  DParamMax=[]  NParamMin=[]  NParamMax=[]  KbParamMin=[]  KbParamMax=[]  KtParamMin=[]  KtParamMax=[]  KbOutMin=[]  KbOutMax=[]  KtOutMin=[]  KtOutMax=[]  IntegratorOutMin=[]  IntegratorOutMax=[]  FilterOutMin=[]  FilterOutMax=[]  SumI1OutMin=[]  SumI1OutMax=[]  SumI2OutMin=[]  SumI2OutMax=[]  SumI3OutMin=[]  SumI3OutMax=[]  SumI4OutMin=[]  SumI4OutMax=[]  SumDOutMin=[]  SumDOutMax=[]  DifferentiatorOutMin=[]  DifferentiatorOutMax=[]  FilterDiffOutCoefMin=[]  FilterDiffOutCoefMax=[]  ReciprocalOutMin=[]  ReciprocalOutMax=[]  SumDenOutMin=[]  SumDenOutMax=[]  SumNumOutMin=[]  SumNumOutMax=[]  DivideOutMin=[]  DivideOutMax=[]  UdiffTsProdOutMin=[]  UdiffTsProdOutMax=[]  NTsProdOutMin=[]  NTsProdOutMax=[]  UintegralTsProdOutMin=[]  UintegralTsProdOutMax=[]  UngainTsProdOutMin=[]  UngainTsProdOutMax=[]  ClampingZeroOutDataTypeStr=Inherit: Inherit via back propagation  ClampingZeroOutMin=[]  ClampingZeroOutMax=[]  FilterDenConstantOutDataTypeStr=Inherit: Inherit via back propagation  FilterDenConstantOutMin=[]  FilterDenConstantOutMax=[]  PCopyOutDataTypeStr=Inherit: Inherit via back propagation  PCopyOutMin=[]  PCopyOutMax=[]  NCopyOutDataTypeStr=Inherit: Inherit via back propagation  NCopyOutMin=[]  NCopyOutMax=[]  IntegratorContinuousStateAttributes=''  IntegratorStateMustResolveToSignalObject=off  IntegratorRTWStateStorageClass=Auto  FilterContinuousStateAttributes=''  FilterStateMustResolveToSignalObject=off  FilterRTWStateStorageClass=Auto  ParallelPVariant=InternalParameters  IdealPVariant=Disabled  IVariant=InternalParameters  DVariant=Disabled  IntegratorVariant=Discrete  SatVariant=Enabled  AWVariant=BackCalculation  PCopyVariant=Disabled  TRVariant=Disabled  FdbkBlocksVariant=Forward  IdealPFdbkVariant=Disabled  SatFdbkVariant=Disabled  DerivativeFilterVariant=Disabled  NVariant=Disabled  NCopyVariant=Disabled_SignalSpec  FilterICVariant=Disabled  IntegratorICVariant=InternalICs  ExternalResetVariant=Disabled  TRSumVariant=Passthrough  SumFdbkVariant=Disabled  SumVariant=Sum_PI  TsampFilterVariant=InternalTs  TsampNgainVariant=Passthrough  TsampIntegralVariant=Disabled_SignalSpec  ExternalSaturationOutDataTypeStr=Inherit: Same as second input  DerivativeSourceVariant=Disabled  PreIntVariant=InternalPreInt
  VdcF1 : InportShadow  Port=2
  d-axis current PI : slpidlib/PID Controller  Controller=PI  Form=Parallel  TimeDomain=Discrete-time  UseExternalTs=off  SampleTime=Tsc  IntegratorMethod=Forward Euler  FilterMethod=Forward Euler  ControllerParametersSource=internal  P=Kp_id  I=Ki_id  UseKiTs=off  D=0  UseExternalDerivativeSource=off  N=100  UseFilter=on  TunerSelectOption=Transfer Function Based (PID Tuner App)  InitialConditionSource=internal  InitialConditionForIntegrator=0  InitialConditionForFilter=0  DifferentiatorICPrevScaledInput=0  ExternalReset=none  TrackingMode=off  Kt=1  LimitOutput=on  SatLimitsSource=internal  UpperSaturationLimit=Req*1*10  LowerSaturationLimit=-Req*1*10  LinearizeAsGain=on  AntiWindupMode=back-calculation  Kb=1000  LimitIntegrator=off  UpperIntegratorSaturationLimit=inf  LowerIntegratorSaturationLimit=-inf  POutMin=[]  POutMax=[]  IOutMin=[]  IOutMax=[]  DOutMin=[]  DOutMax=[]  NOutMin=[]  NOutMax=[]  SumOutMin=[]  SumOutMax=[]  SaturationOutMin=[]  SaturationOutMax=[]  PParamMin=[]  PParamMax=[]  IParamMin=[]  IParamMax=[]  DParamMin=[]  DParamMax=[]  NParamMin=[]  NParamMax=[]  KbParamMin=[]  KbParamMax=[]  KtParamMin=[]  KtParamMax=[]  KbOutMin=[]  KbOutMax=[]  KtOutMin=[]  KtOutMax=[]  IntegratorOutMin=[]  IntegratorOutMax=[]  FilterOutMin=[]  FilterOutMax=[]  SumI1OutMin=[]  SumI1OutMax=[]  SumI2OutMin=[]  SumI2OutMax=[]  SumI3OutMin=[]  SumI3OutMax=[]  SumI4OutMin=[]  SumI4OutMax=[]  SumDOutMin=[]  SumDOutMax=[]  DifferentiatorOutMin=[]  DifferentiatorOutMax=[]  FilterDiffOutCoefMin=[]  FilterDiffOutCoefMax=[]  ReciprocalOutMin=[]  ReciprocalOutMax=[]  SumDenOutMin=[]  SumDenOutMax=[]  SumNumOutMin=[]  SumNumOutMax=[]  DivideOutMin=[]  DivideOutMax=[]  UdiffTsProdOutMin=[]  UdiffTsProdOutMax=[]  NTsProdOutMin=[]  NTsProdOutMax=[]  UintegralTsProdOutMin=[]  UintegralTsProdOutMax=[]  UngainTsProdOutMin=[]  UngainTsProdOutMax=[]  ClampingZeroOutDataTypeStr=Inherit: Inherit via back propagation  ClampingZeroOutMin=[]  ClampingZeroOutMax=[]  FilterDenConstantOutDataTypeStr=Inherit: Inherit via back propagation  FilterDenConstantOutMin=[]  FilterDenConstantOutMax=[]  PCopyOutDataTypeStr=Inherit: Inherit via back propagation  PCopyOutMin=[]  PCopyOutMax=[]  NCopyOutDataTypeStr=Inherit: Inherit via back propagation  NCopyOutMin=[]  NCopyOutMax=[]  IntegratorContinuousStateAttributes=''  IntegratorStateMustResolveToSignalObject=off  IntegratorRTWStateStorageClass=Auto  FilterContinuousStateAttributes=''  FilterStateMustResolveToSignalObject=off  FilterRTWStateStorageClass=Auto  ParallelPVariant=InternalParameters  IdealPVariant=Disabled  IVariant=InternalParameters  DVariant=Disabled  IntegratorVariant=Discrete  SatVariant=Enabled  AWVariant=BackCalculation  PCopyVariant=Disabled  TRVariant=Disabled  FdbkBlocksVariant=Forward  IdealPFdbkVariant=Disabled  SatFdbkVariant=Disabled  DerivativeFilterVariant=Disabled  NVariant=Disabled  NCopyVariant=Disabled_SignalSpec  FilterICVariant=Disabled  IntegratorICVariant=InternalICs  ExternalResetVariant=Disabled  TRSumVariant=Passthrough  SumFdbkVariant=Disabled  SumVariant=Sum_PI  TsampFilterVariant=InternalTs  TsampNgainVariant=Passthrough  TsampIntegralVariant=Disabled_SignalSpec  ExternalSaturationOutDataTypeStr=Inherit: Same as second input  DerivativeSourceVariant=Disabled  PreIntVariant=InternalPreInt
  dq->abc : eeTransforms/Inverse Park Transform  AxisAlignment=Q-axis  PowerInvariant=off
  i_q* : Constant  Value=0
  idF1 : InportShadow  Port=5
  iqF1 : InportShadow  Port=7
  omega1 : InportShadow  Port=3
  "p.u. -> V1" : Gain  Gain=Vt1base*N
  q-axis current PI : slpidlib/PID Controller  Controller=PI  Form=Parallel  TimeDomain=Discrete-time  UseExternalTs=off  SampleTime=Tsc  IntegratorMethod=Forward Euler  FilterMethod=Forward Euler  ControllerParametersSource=internal  P=Kp_iq  I=Ki_iq  UseKiTs=off  D=0  UseExternalDerivativeSource=off  N=100  UseFilter=on  TunerSelectOption=Transfer Function Based (PID Tuner App)  InitialConditionSource=internal  InitialConditionForIntegrator=0  InitialConditionForFilter=0  DifferentiatorICPrevScaledInput=0  ExternalReset=none  TrackingMode=off  Kt=1  LimitOutput=on  SatLimitsSource=internal  UpperSaturationLimit=Req*1*10  LowerSaturationLimit=-Req*1*10  LinearizeAsGain=on  AntiWindupMode=back-calculation  Kb=1000  LimitIntegrator=off  UpperIntegratorSaturationLimit=inf  LowerIntegratorSaturationLimit=-inf  POutMin=[]  POutMax=[]  IOutMin=[]  IOutMax=[]  DOutMin=[]  DOutMax=[]  NOutMin=[]  NOutMax=[]  SumOutMin=[]  SumOutMax=[]  SaturationOutMin=[]  SaturationOutMax=[]  PParamMin=[]  PParamMax=[]  IParamMin=[]  IParamMax=[]  DParamMin=[]  DParamMax=[]  NParamMin=[]  NParamMax=[]  KbParamMin=[]  KbParamMax=[]  KtParamMin=[]  KtParamMax=[]  KbOutMin=[]  KbOutMax=[]  KtOutMin=[]  KtOutMax=[]  IntegratorOutMin=[]  IntegratorOutMax=[]  FilterOutMin=[]  FilterOutMax=[]  SumI1OutMin=[]  SumI1OutMax=[]  SumI2OutMin=[]  SumI2OutMax=[]  SumI3OutMin=[]  SumI3OutMax=[]  SumI4OutMin=[]  SumI4OutMax=[]  SumDOutMin=[]  SumDOutMax=[]  DifferentiatorOutMin=[]  DifferentiatorOutMax=[]  FilterDiffOutCoefMin=[]  FilterDiffOutCoefMax=[]  ReciprocalOutMin=[]  ReciprocalOutMax=[]  SumDenOutMin=[]  SumDenOutMax=[]  SumNumOutMin=[]  SumNumOutMax=[]  DivideOutMin=[]  DivideOutMax=[]  UdiffTsProdOutMin=[]  UdiffTsProdOutMax=[]  NTsProdOutMin=[]  NTsProdOutMax=[]  UintegralTsProdOutMin=[]  UintegralTsProdOutMax=[]  UngainTsProdOutMin=[]  UngainTsProdOutMax=[]  ClampingZeroOutDataTypeStr=Inherit: Inherit via back propagation  ClampingZeroOutMin=[]  ClampingZeroOutMax=[]  FilterDenConstantOutDataTypeStr=Inherit: Inherit via back propagation  FilterDenConstantOutMin=[]  FilterDenConstantOutMax=[]  PCopyOutDataTypeStr=Inherit: Inherit via back propagation  PCopyOutMin=[]  PCopyOutMax=[]  NCopyOutDataTypeStr=Inherit: Inherit via back propagation  NCopyOutMin=[]  NCopyOutMax=[]  IntegratorContinuousStateAttributes=''  IntegratorStateMustResolveToSignalObject=off  IntegratorRTWStateStorageClass=Auto  FilterContinuousStateAttributes=''  FilterStateMustResolveToSignalObject=off  FilterRTWStateStorageClass=Auto  ParallelPVariant=InternalParameters  IdealPVariant=Disabled  IVariant=InternalParameters  DVariant=Disabled  IntegratorVariant=Discrete  SatVariant=Enabled  AWVariant=BackCalculation  PCopyVariant=Disabled  TRVariant=Disabled  FdbkBlocksVariant=Forward  IdealPFdbkVariant=Disabled  SatFdbkVariant=Disabled  DerivativeFilterVariant=Disabled  NVariant=Disabled  NCopyVariant=Disabled_SignalSpec  FilterICVariant=Disabled  IntegratorICVariant=InternalICs  ExternalResetVariant=Disabled  TRSumVariant=Passthrough  SumFdbkVariant=Disabled  SumVariant=Sum_PI  TsampFilterVariant=InternalTs  TsampNgainVariant=Passthrough  TsampIntegralVariant=Disabled_SignalSpec  ExternalSaturationOutDataTypeStr=Inherit: Same as second input  DerivativeSourceVariant=Disabled  PreIntVariant=InternalPreInt
  SR : Outport  VectorParamsAs1DForOutWhenUnconnected=off
  wires:
  Sum5/1 -> q-axis current PI/1
  Vdc PI2/1 -> Sum1/1
  theta/1 -> dq->abc/2
  Sum4/1 -> Mux4/2
  Vdc/1 -> Sum3/1
  d-axis current PI/1 -> Sum2/2
  Subtract2/1 -> Sum2/1
  Sum2/1 -> Mux4/1
  Sum1/1 -> d-axis current PI/1
  --> p.u./1 -> Vdc PI2/1
  Avoid division by zero/1 -> PWM generator/2
  Divide4/1 -> "Leq "/1
  Leq/1 -> Subtract2/2
  i_q*/1 -> Sum5/1
  PWM generator/1 -> SR/1
  omega/1 -> Divide3/1
  q-axis current PI/1 -> Sum4/1
  Mux4/1 -> "p.u. -> V1"/1
  Divide3/1 -> Leq/1
  Mux1/1 -> dq->abc/1
  Constant1/1 -> Mux1/2
  "Leq "/1 -> Sum4/2
  idF/1 -> Divide4/2
  PWM generator/2 -> Terminator/1
  VdcF/1 -> Sum3/2
  dq->abc/1 -> PWM generator/1
  "p.u. -> V1"/1 -> Mux1/1
  Sum3/1 -> --> p.u./1
  iqF/1 -> Divide3/2
  Vg/1 -> Subtract2/1
  iqF1/1 -> Sum5/2
  omega1/1 -> Divide4/1
  idF1/1 -> Sum1/2
  VdcF1/1 -> Avoid division by zero/1
